simulink model "A3Model"  (R2017a)
settings: Solver=VariableStepAuto  StartTime=0.0  StopTime=10  RelTol=1e-3
undefined symbols (not defined in the file or in its folder): MassKg
libraries: simulink x1
settings Model: Creator=Ivan  LastModifiedBy=Ivan

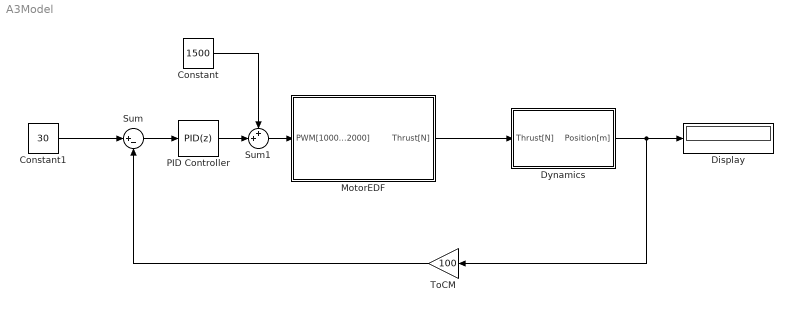
== system A3Model ==
  Constant : Constant  Value=1500
  Constant1 : Constant  Value=30
  Display : Display
  Dynamics : Subsystem
  MotorEDF : Subsystem
  PID Controller : simulink/Continuous/PID Controller  Controller=PID  TimeDomain=Discrete-time  SampleTime=0.02  IntegratorMethod=Forward Euler  FilterMethod=Forward Euler  Form=Parallel  UseFilter=on  ControllerParametersSource=internal  P=1  I=0.045  D=5  N=90  InitialConditionSource=internal  InitialConditionForIntegrator=0  InitialConditionForFilter=0  ExternalReset=none  LimitOutput=off  UpperSaturationLimit=inf  LowerSaturationLimit=-inf  LinearizeAsGain=on  AntiWindupMode=none  Kb=1  TrackingMode=off  Kt=1  PParamMin=[]  PParamMax=[]  IParamMin=[]  IParamMax=[]  DParamMin=[]  DParamMax=[]  NParamMin=[]  NParamMax=[]  KbParamMin=[]  KbParamMax=[]  KtParamMin=[]  KtParamMax=[]  POutMin=[]  POutMax=[]  IOutMin=[]  IOutMax=[]  DOutMin=[]  DOutMax=[]  NOutMin=[]  NOutMax=[]  KbOutMin=[]  KbOutMax=[]  KtOutMin=[]  KtOutMax=[]  IntegratorOutMin=[]  IntegratorOutMax=[]  FilterOutMin=[]  FilterOutMax=[]  SumOutMin=[]  SumOutMax=[]  SumI1OutMin=[]  SumI1OutMax=[]  SumI2OutMin=[]  SumI2OutMax=[]  SumI3OutMin=[]  SumI3OutMax=[]  SumDOutMin=[]  SumDOutMax=[]  SaturationOutMin=[]  SaturationOutMax=[]  IntegratorContinuousStateAttributes=''  IntegratorStateMustResolveToSignalObject=off  IntegratorRTWStateStorageClass=Auto  FilterContinuousStateAttributes=''  FilterStateMustResolveToSignalObject=off  FilterRTWStateStorageClass=Auto  DifferentiatorICPrevScaledInput=0  DifferentiatorOutMin=[]  DifferentiatorOutMax=[]  InitialConditionSetting=State (most efficient)
  Sum : Sum  Inputs=|+-
  Sum1 : Sum  Inputs=++|
  ToCM : Gain  Gain=100
  wires:
  MotorEDF/1(Thrust[N]) -> Dynamics/1(Thrust[N])
  Dynamics/1(Position[m]) -> ToCM/1, Display/1
  ToCM/1 -> Sum/2
  Sum/1 -> PID Controller/1
  Constant1/1 -> Sum/1
  PID Controller/1 -> Sum1/2
  Sum1/1 -> MotorEDF/1(PWM[1000...2000])
  Constant/1 -> Sum1/1

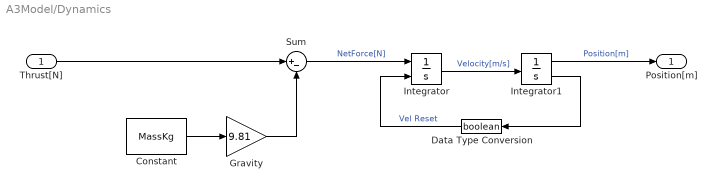
== system A3Model/Dynamics ==
  Thrust[N] : Inport
  Constant : Constant  Value=MassKg
  Data Type Conversion : DataTypeConversion  OutDataTypeStr=boolean
  Gravity : Gain  Gain=9.81
  Integrator : Integrator  ExternalReset=rising
  Integrator1 : Integrator  InitialCondition=0.3  LimitOutput=on  UpperSaturationLimit=3  LowerSaturationLimit=-3  ShowSaturationPort=on
  Sum : Sum  Inputs=|+-
  Position[m] : Outport
  wires:
  Data Type Conversion/1 -> Integrator/2  "Vel Reset"
  Integrator1/2 -> Data Type Conversion/1
  Integrator1/1 -> Position[m]/1  "Position[m]"
  Constant/1 -> Gravity/1
  Gravity/1 -> Sum/2
  Thrust[N]/1 -> Sum/1
  Sum/1 -> Integrator/1  "NetForce[N]"
  Integrator/1 -> Integrator1/1  "Velocity[m/s]"

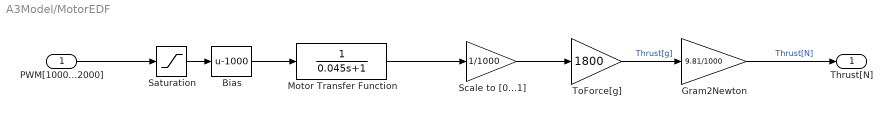
== system A3Model/MotorEDF ==
  PWM[1000...2000] : Inport
  Bias : Bias  Bias=-1000
  Gram2Newton : Gain  Gain=9.81/1000
  Motor Transfer Function : TransferFcn  Denominator=[0.045 1]
  Saturation : Saturate  UpperLimit=2000  LowerLimit=1000
  Scale to [0...1] : Gain  Gain=1/1000
  ToForce[g] : Gain  Gain=1800
  Thrust[N] : Outport
  wires:
  Saturation/1 -> Bias/1
  PWM[1000...2000]/1 -> Saturation/1
  Gram2Newton/1 -> Thrust[N]/1  "Thrust[N]"
  Scale to [0...1]/1 -> ToForce[g]/1
  Motor Transfer Function/1 -> Scale to [0...1]/1
  Bias/1 -> Motor Transfer Function/1
  ToForce[g]/1 -> Gram2Newton/1  "Thrust[g]"
